simulink model "obs_tests"  (R2025b)
settings: Solver=VariableStepAuto  StartTime=0.0  StopTime=5  RelTol=1e-3
values from neighbouring files (symbols this model uses):
  A = [-B/J,    Kt/J ... (first row only)    [demo.m]
  A_d = [-B/J,    Kt/J ... (first row only)    [demo.m]
  Ae = A - L*C    [demo.m]
  B_ss = [0; 1/La]    [demo.m]
  Be = [B_ss, L]    [demo.m]
  C = [1, 0]    [demo.m]
  Ce = eye(2)    [demo.m]
  De = zeros(2,2)    [demo.m]
  V = 24    [demo.m]
libraries: simulink x9
settings Model: Creator=wepi  LastModifiedBy=wepi

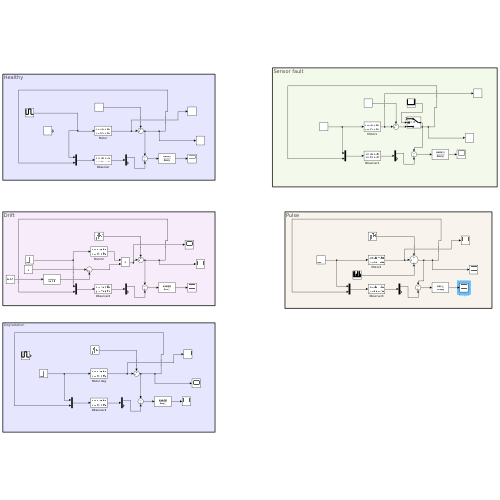
[thumbnail: Simulink's stored preview of the top-level diagram]
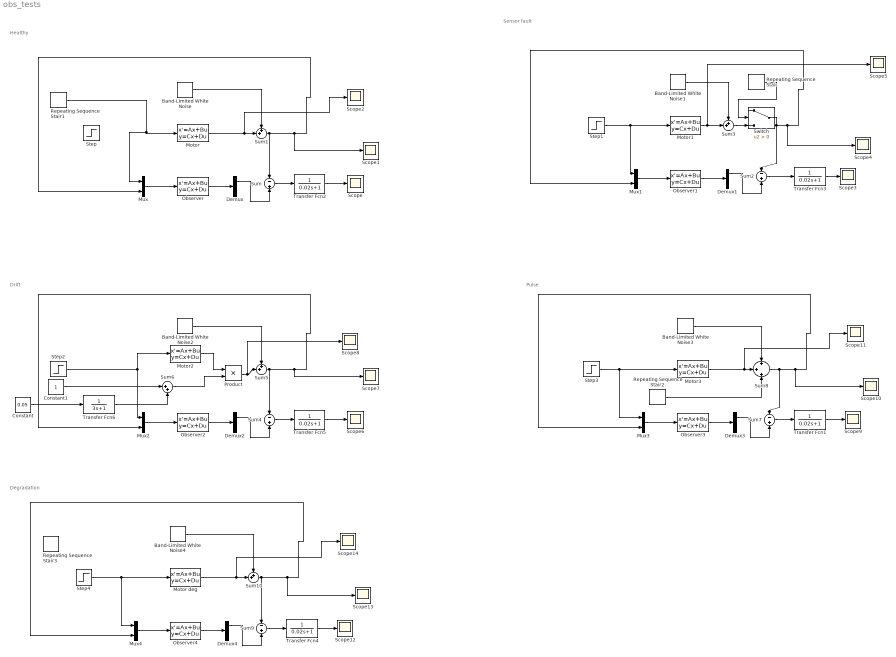
== system obs_tests ==
  note: Degradation
  note: Pulse
  note: Drift
  note: Sensor fault
  note: Healthy
  Band-Limited White Noise{,1..4} (5 alike) : simulink/Sources/Band-Limited White Noise  Cov=[5.1e-4]  Ts=1e-4  seed=[23341]
  Constant : Constant  Value=0.05
  Constant1 : Constant
  Demux{,1..4} (5 alike) : Demux  Outputs=2
  Motor{,1..3} (4 alike) : StateSpace  A=A  B=B_ss  C=C  D=0  InitialCondition=0
  Motor deg : StateSpace  A=A_d  B=B_ss  C=C  D=0  InitialCondition=0
  Mux{,1..4} (5 alike) : Mux  Inputs=2
  Observer{,1..4} (5 alike) : StateSpace  A=Ae  B=Be  C=Ce  D=De  InitialCondition=0
  Product : Product
  Repeating Sequence Stair : simulink/Sources/Repeating Sequence Stair  OutValues=[0 0 0 0 0 0 0 0 0 0 0 0 0 0 0 0 0 0 0 10 0].'  tsamp=0.1  OutMin=[]  OutMax=[]  OutDataTypeStr=double  OutputDataTypeScalingMode=double  OutDataType=fixdt(0,8)  ConRadixGroup=Best Precision: Vector-wise  OutScaling=2^-12
  Repeating Sequence Stair1 : simulink/Sources/Repeating Sequence Stair  OutValues=[24 27 24].'  tsamp=2  OutMin=[]  OutMax=[]  OutDataTypeStr=double  OutputDataTypeScalingMode=double  OutDataType=fixdt(0,8)  ConRadixGroup=Best Precision: Vector-wise  OutScaling=2^-12
  Repeating Sequence Stair2 : simulink/Sources/Repeating Sequence Stair  OutValues=[0 0 0 0 2 0 0 0 0 1 0 0 0 0 2 0 0 0 0 2 0 0 0 0 1].'  tsamp=0.1  OutMin=[]  OutMax=[]  OutDataTypeStr=double  OutputDataTypeScalingMode=double  OutDataType=fixdt(0,8)  ConRadixGroup=Best Precision: Vector-wise  OutScaling=2^-12
  Repeating Sequence Stair3 : simulink/Sources/Repeating Sequence Stair  OutValues=[24 27 24].'  tsamp=2  OutMin=[]  OutMax=[]  OutDataTypeStr=double  OutputDataTypeScalingMode=double  OutDataType=fixdt(0,8)  ConRadixGroup=Best Precision: Vector-wise  OutScaling=2^-12
  Scope{,1..14} (15 alike) : Scope
      Scope settings: ActiveDisplayYMinimum=-0.72610573986208593  ActiveDisplayYMaximum=1.1678760313251231
      Scope1 settings: ActiveDisplayYMinimum=-38.403685909936847  ActiveDisplayYMaximum=264.2167855090695
      Scope10 settings: ActiveDisplayYMinimum=-38.403685909936847  ActiveDisplayYMaximum=264.2167855090695  DataLoggingVariableName=ScopeData9
      Scope11 settings: ActiveDisplayYMinimum=-28.225398175178814  ActiveDisplayYMaximum=254.02858357660938  DataLoggingVariableName=ScopeData10
      Scope12 settings: ActiveDisplayYMinimum=-0.803803301939585  ActiveDisplayYMaximum=1.4123280102590092  DataLoggingVariableName=ScopeData12
      Scope13 settings: ActiveDisplayYMinimum=-38.403685909936847  ActiveDisplayYMaximum=264.2167855090695  DataLoggingVariableName=ScopeData13
      Scope14 settings: ActiveDisplayYMinimum=-28.225398175178814  ActiveDisplayYMaximum=254.02858357660938  DataLoggingVariableName=ScopeData14
      Scope2 settings: ActiveDisplayYMinimum=-28.225398175178814  ActiveDisplayYMaximum=254.02858357660938  DataLoggingVariableName=ScopeData2
      Scope3 settings: ActiveDisplayYMinimum=-21.178946469637097  ActiveDisplayYMaximum=37.765082799994794  DataLoggingVariableName=ScopeData3
      Scope4 settings: ActiveDisplayYMinimum=-46.249544242775315  ActiveDisplayYMaximum=247.3311083298272  DataLoggingVariableName=ScopeData4
      Scope5 settings: ActiveDisplayYMinimum=-28.225398175178814  ActiveDisplayYMaximum=254.02858357660938  DataLoggingVariableName=ScopeData5
      Scope6 settings: ActiveDisplayYMinimum=-0.75810166052402184  ActiveDisplayYMaximum=0.1637336183017532  DataLoggingVariableName=ScopeData6
      Scope7 settings: ActiveDisplayYMinimum=-75.950514670016162  ActiveDisplayYMaximum=288.29195117236105  DataLoggingVariableName=ScopeData7
      Scope8 settings: ActiveDisplayYMinimum=-30.514827546530736  ActiveDisplayYMaximum=274.63344791877671  DataLoggingVariableName=ScopeData8
      Scope9 settings: ActiveDisplayYMinimum=-0.44905788790208173  ActiveDisplayYMaximum=0.25576448097686838  DataLoggingVariableName=ScopeData11
  Step{,1..4} (5 alike) : Step  Time=0.1  After=V  SampleTime=0
  Sum{,2,4,7,9} (5 alike) : Sum  Inputs=-|+
  Sum{1,3,5,10} (4 alike) : Sum  Inputs=++|
  Sum6 : Sum  Inputs=|++
  Sum8 : Sum  Inputs=+|+|+
  Switch : Switch  Criteria=u2 > Threshold  SaturateOnIntegerOverflow=off  InputSameDT=off
  Transfer Fcn{1..5} (5 alike) : TransferFcn  Denominator=[0.02 1]
  Transfer Fcn6 : TransferFcn  Denominator=[3 1]
  wires:
  Mux/1 -> Observer/1
  Observer/1 -> Demux/1
  Demux/1 -> Sum/2
  Sum/1 -> Transfer Fcn2/1
  Motor/1 -> Scope2/1, Sum1/2
  Band-Limited White Noise/1 -> Sum1/1
  Sum1/1 -> Scope1/1, Mux/2, Sum/1
  Mux1/1 -> Observer1/1
  Demux1/1 -> Sum2/2
  Switch/1 -> Scope4/1, Mux1/2, Sum2/1
  Motor1/1 -> Scope5/1, Sum3/2
  Observer1/1 -> Demux1/1
  Step1/1 -> Mux1/1, Motor1/1
  Band-Limited White Noise1/1 -> Sum3/1
  Sum2/1 -> Transfer Fcn3/1
  Transfer Fcn2/1 -> Scope/1
  Transfer Fcn3/1 -> Scope3/1
  Sum3/1 -> Switch/3
  Repeating Sequence Stair/1 -> Switch/2
  Mux2/1 -> Observer2/1
  Demux2/1 -> Sum4/2
  Sum5/1 -> Scope7/1, Mux2/2, Sum4/1
  Motor2/1 -> Product/1
  Observer2/1 -> Demux2/1
  Transfer Fcn5/1 -> Scope6/1
  Step2/1 -> Mux2/1, Motor2/1
  Band-Limited White Noise2/1 -> Sum5/1
  Sum4/1 -> Transfer Fcn5/1
  Constant/1 -> Transfer Fcn6/1
  Sum6/1 -> Product/2
  Transfer Fcn6/1 -> Sum6/2
  Constant1/1 -> Sum6/1
  Product/1 -> Scope8/1, Sum5/2
  Repeating Sequence Stair1/1 -> Mux/1, Motor/1
  Mux3/1 -> Observer3/1
  Observer3/1 -> Demux3/1
  Band-Limited White Noise3/1 -> Sum8/1
  Sum8/1 -> Scope10/1, Mux3/2, Sum7/1
  Sum7/1 -> Transfer Fcn1/1
  Transfer Fcn1/1 -> Scope9/1
  Demux3/1 -> Sum7/2
  Motor3/1 -> Scope11/1, Sum8/2
  Step3/1 -> Mux3/1, Motor3/1
  Repeating Sequence Stair2/1 -> Sum8/3
  Mux4/1 -> Observer4/1
  Observer4/1 -> Demux4/1
  Band-Limited White Noise4/1 -> Sum10/1
  Sum10/1 -> Scope13/1, Mux4/2, Sum9/1
  Sum9/1 -> Transfer Fcn4/1
  Transfer Fcn4/1 -> Scope12/1
  Demux4/1 -> Sum9/2
  Motor deg/1 -> Scope14/1, Sum10/2
  Step4/1 -> Mux4/1, Motor deg/1
